simulink model "Nodos_primer_control"  (R2019a)
settings: Solver=VariableStepAuto  StartTime=0.0  StopTime=50  RelTol=1e-3
values from neighbouring files (symbols this model uses):
  hdis = hdis'    [programa_nodos.m]
  tm = 0.5    [programa_nodos.m]
undefined symbols (not defined in the file or in its folder): adis, bdis, cdis
settings Model: Creator=Alejoxbg  LastModifiedBy=Alejoxbg

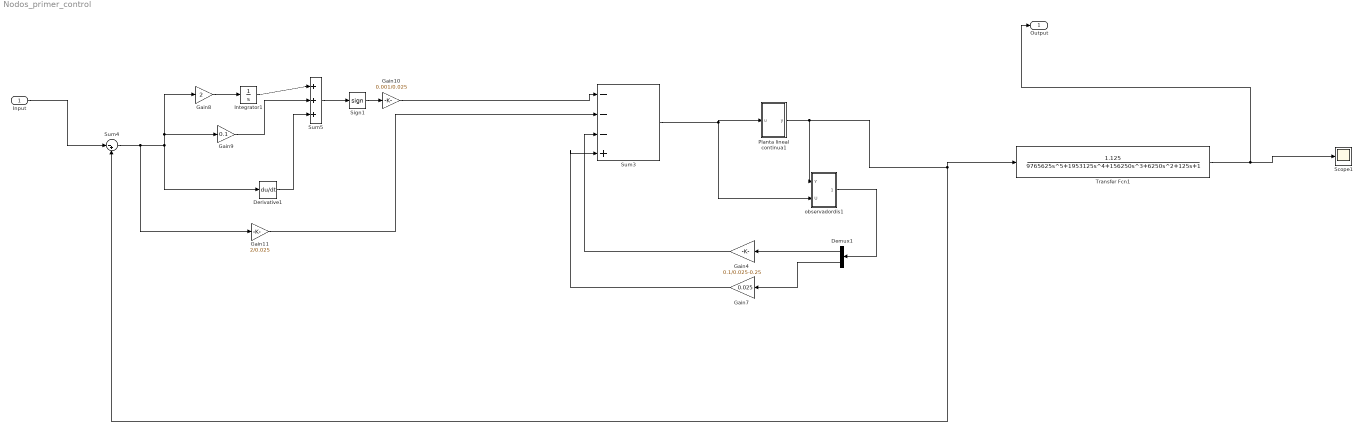
== system Nodos_primer_control ==
  Input : Inport
  Demux1 : Demux  Outputs=2
  Derivative1 : Derivative
  Gain10 : Gain  Gain=0.001/0.025
  Gain11 : Gain  Gain=2/0.025
  Gain4 : Gain  Gain=0.1/0.025-0.25
  Gain7 : Gain  Gain=0.025
  Gain8 : Gain  Gain=2
  Gain9 : Gain  Gain=0.1
  Integrator1 : Integrator
  Planta lineal continua1 : Subsystem
  Scope1 : Scope
  Sign1 : Signum  ZeroCross=off
  Sum3 : Sum  Inputs=|---+
  Sum4 : Sum  Inputs=|-+
  Sum5 : Sum  Inputs=|+++
  Transfer Fcn1 : TransferFcn  Numerator=[1.125]  Denominator="[9765625     1953125      156250        6250         125           1]"
  observadordis1 : Subsystem
  Output : Outport
  wires:
  Gain11/1 -> Sum3/2
  Gain8/1 -> Integrator1/1
  Gain7/1 -> Sum3/4
  Gain4/1 -> Sum3/3
  Sum5/1 -> Sign1/1
  Demux1/2 -> Gain7/1
  Gain9/1 -> Sum5/2
  Sum3/1 -> Planta lineal continua1/1(u), observadordis1/2(U)
  Integrator1/1 -> Sum5/1
  Derivative1/1 -> Sum5/3
  observadordis1/1(xgorro) -> Demux1/1
  Planta lineal continua1/1(y) -> observadordis1/1(Y), Sum4/2, Transfer Fcn1/1
  Sum4/1 -> Gain11/1, Derivative1/1, Gain8/1, Gain9/1
  Demux1/1 -> Gain4/1
  Gain10/1 -> Sum3/1
  Sign1/1 -> Gain10/1
  Transfer Fcn1/1 -> Output/1, Scope1/1
  Input/1 -> Sum4/1

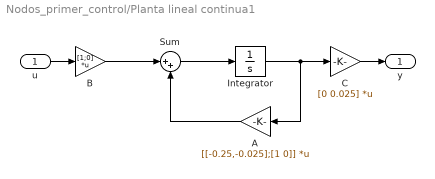
== system Nodos_primer_control/Planta lineal continua1 ==
  u : Inport
  A : Gain  Gain=[[-0.25,-0.025];[1 0]]  Multiplication=Matrix(K*u) (u vector)
  B : Gain  Gain=[1;0]  Multiplication=Matrix(K*u) (u vector)
  C : Gain  Gain=[0 0.025]  Multiplication=Matrix(K*u) (u vector)
  Integrator : Integrator
  Sum : Sum  Inputs=|++
  y : Outport
  wires:
  C/1 -> y/1
  u/1 -> B/1
  Integrator/1 -> A/1, C/1
  A/1 -> Sum/2
  Sum/1 -> Integrator/1
  B/1 -> Sum/1

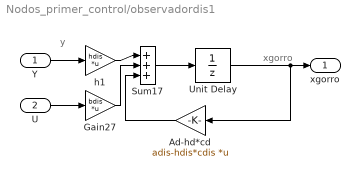
== system Nodos_primer_control/observadordis1 ==
  note: xgorro
  note: y
  Y : Inport
  U : Inport  Port=2
  Ad-hd*cd : Gain  Gain=adis-hdis*cdis  Multiplication=Matrix(K*u) (u vector)  SampleTime=tm
  Gain27 : Gain  Gain=bdis  Multiplication=Matrix(K*u) (u vector)  SampleTime=tm
  Sum17 : Sum  Inputs=|+++
  Unit Delay : UnitDelay  SampleTime=tm  HasFrameUpgradeWarning=on
  h1 : Gain  Gain=hdis  Multiplication=Matrix(K*u) (u vector)  SampleTime=tm
  xgorro : Outport
  wires:
  Sum17/1 -> Unit Delay/1
  h1/1 -> Sum17/1
  Unit Delay/1 -> Ad-hd*cd/1, xgorro/1
  Ad-hd*cd/1 -> Sum17/3
  Gain27/1 -> Sum17/2
  Y/1 -> h1/1
  U/1 -> Gain27/1
